simulink model "pmsm_position_control"  (R2024b)
settings: Solver=VariableStepAuto  StartTime=0.0  StopTime=10.0  RelTol=1e-3
values from neighbouring files (symbols this model uses):
  Ki_pos = 200.0    (= 200)    [simulate_surface_pmsm_foc.m]    (also in step4_build_position_loop.m = 78.5398163397; step5d_position_control.m = 78.5398163397)
  Kp_pos = 5.0    (= 5)    [simulate_surface_pmsm_foc.m]    (also in step4_build_position_loop.m = 31.4159265359; step5d_position_control.m = 31.4159265359)
  omega_max = 300    [step5b_current_control.m]    (also in step5c_speed_control.m; step5d_position_control.m)
settings Model: Creator=Lee  LastModifiedBy=Lee

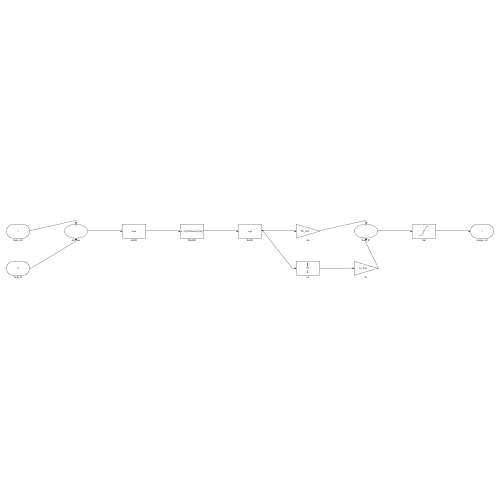
[thumbnail: Simulink's stored preview of the top-level diagram]
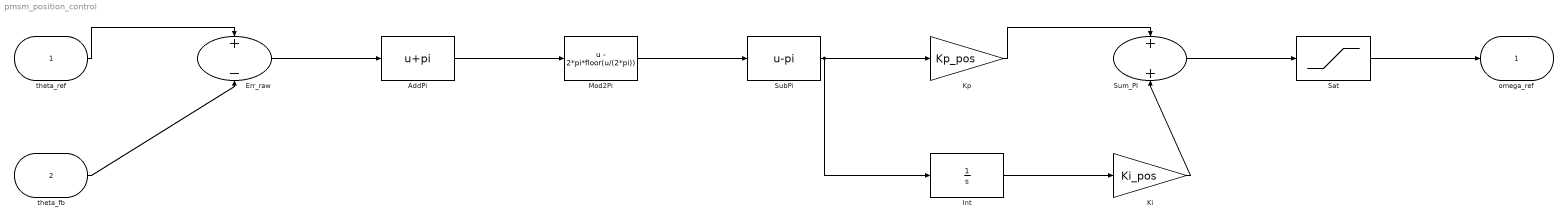
== system pmsm_position_control ==
  theta_ref : Inport
  theta_fb : Inport  Port=2
  AddPi : Fcn  Expr=u+pi
  Err_raw : Sum  Inputs=+-
  Int : Integrator
  Ki : Gain  Gain=Ki_pos
  Kp : Gain  Gain=Kp_pos
  Mod2Pi : Fcn  Expr=u - 2*pi*floor(u/(2*pi))
  Sat : Saturate  UpperLimit=omega_max  LowerLimit=-omega_max
  SubPi : Fcn  Expr=u-pi
  Sum_PI : Sum
  omega_ref : Outport
  wires:
  theta_ref/1 -> Err_raw/1
  theta_fb/1 -> Err_raw/2
  Err_raw/1 -> AddPi/1
  AddPi/1 -> Mod2Pi/1
  Mod2Pi/1 -> SubPi/1
  SubPi/1 -> Kp/1, Int/1
  Int/1 -> Ki/1
  Kp/1 -> Sum_PI/1
  Ki/1 -> Sum_PI/2
  Sum_PI/1 -> Sat/1
  Sat/1 -> omega_ref/1
